simulink model "RADTRANS002"  (R2020b)
settings: Solver=VariableStepAuto  StartTime=0.0  StopTime=10.0  RelTol=1e-3
undefined symbols (not defined in the file): Line_110_C, Line_110_L, Line_110_R, Line_220_C, Line_220_L, Line_220_R, Line_35_C, Line_35_L, Line_35_R, Line_6_L, Line_6_R, Sys_f_Hz, Sys_V_net_kV, Tr_110_35_L_pu, Tr_110_35_R_pu, Tr_110_35_Sn_VA, Tr_110_35_V_HV_kV, Tr_110_35_V_LV_kV, Tr_110_6_L_pu, Tr_110_6_R_pu, Tr_110_6_Sn_VA, Tr_110_6_V_HV_kV, Tr_110_6_V_LV_kV, Tr_220_110_L_pu, Tr_220_110_R_pu, Tr_220_110_Sn_VA, Tr_220_110_V_HV_kV, Tr_220_110_V_LV_kV, Tr_35_04_L_pu, Tr_35_04_R_pu, Tr_35_04_Sn_VA, Tr_35_04_V_HV_kV, Tr_35_04_V_LV_kV, Tr_6_04_L_pu, Tr_6_04_R_pu, Tr_6_04_Sn_VA, Tr_6_04_V_HV_kV, Tr_6_04_V_LV_kV, Ts_powergui
libraries: dspstat3 x288, powerlib x202, powerlib_meascontrol x72
(part 5 of 7)

== system RADTRANS002/M_IN_Завод_6_1 ==
  Iptg_61 : Display
      settings: Format=bank
  PQptg_61 : Scope  NumInputPorts=2
  "Power0 (3ph, Instantaneous)" : powerlib_meascontrol/Measurements/Power (3ph, Instantaneous)
  Pptg_61 : Display
      settings: Format=bank
  Qptg_61 : Display
      settings: Format=bank
  RMS3 : dspstat3/RMS  run=off  directionMode=Each column  dimension=1  InputProcessing=Columns as channels (frame based)  reset_popup=None
  RMS4 : dspstat3/RMS  run=off  directionMode=Each column  dimension=1  InputProcessing=Columns as channels (frame based)  reset_popup=None
  RMS61 : dspstat3/RMS  run=off  directionMode=Each column  dimension=1  InputProcessing=Columns as channels (frame based)  reset_popup=None
  RMSpt_61 : dspstat3/RMS  run=off  directionMode=Each column  dimension=1  InputProcessing=Columns as channels (frame based)  reset_popup=None
  Real-Ima to Complex : RealImagToComplex
  S : Abs
  SSptg_61 : Scope
  Sptg_61 : Display
      settings: Format=bank
  Three-Phase V-I Measurementpt_61 : powerlib/Measurements/Three-Phase V-I Measurement  VoltageMeasurement=phase-to-ground  SetLabelV=off  LabelV=Vabc  Vpu=off  VpuLL=off  CurrentMeasurement=yes  SetLabelI=off  LabelI=Iabc  Ipu=off  Pbase=100e6  Vbase=500e3  OutputType=Complex  PhasorSimulation=off  PSBequivalent=0
  UIptg_61 : Scope  NumInputPorts=2
  Uptg_61 : Display
      settings: Format=bank
  a : PMIOPort  Side=Right
  b : PMIOPort  Port=2  Side=Right
  c : PMIOPort  Port=3  Side=Right
  A : PMIOPort  Port=4  Side=Left
  B : PMIOPort  Port=5  Side=Left
  C : PMIOPort  Port=6  Side=Left
  tag scope: I_ptg_61=global, P_ptg_61=global, Q_ptg_61=global, S_ptg_61=global, U_ptg_61=global
  wires:
  S/1 -> [S_ptg_61]
  Real-Ima to Complex/1 -> S/1
  [S_ptg_61] -> Sptg_61/1
  [S_ptg_61] -> SSptg_61/1
  [P_ptg_61] -> RMSpt_61/1
  RMSpt_61/1 -> Pptg_61/1
  RMS61/1 -> Qptg_61/1
  [U_ptg_61] -> RMS3/1
  RMS3/1 -> Uptg_61/1
  [P_ptg_61] -> Real-Ima to Complex/1
  [Q_ptg_61] -> RMS61/1
  [I_ptg_61] -> RMS4/1
  RMS4/1 -> Iptg_61/1
  [U_ptg_61] -> UIptg_61/1  "U"
  [P_ptg_61] -> PQptg_61/1  "P"
  [I_ptg_61] -> UIptg_61/2  "I"
  Three-Phase V-I Measurementpt_61/1 -> [U_ptg_61]
  [Q_ptg_61] -> Real-Ima to Complex/2
  Three-Phase V-I Measurementpt_61/2 -> [I_ptg_61]
  [U_ptg_61] -> "Power0 (3ph, Instantaneous)"/1
  [I_ptg_61] -> "Power0 (3ph, Instantaneous)"/2
  "Power0 (3ph, Instantaneous)"/2 -> [Q_ptg_61]
  "Power0 (3ph, Instantaneous)"/1 -> [P_ptg_61]
  [Q_ptg_61] -> PQptg_61/2  "Q"
  connections:
  Three-Phase V-I Measurementpt_61/LConn1 -- A/RConn1
  Three-Phase V-I Measurementpt_61/RConn1 -- a/RConn1
  Three-Phase V-I Measurementpt_61/LConn2 -- B/RConn1
  Three-Phase V-I Measurementpt_61/LConn3 -- C/RConn1
  Three-Phase V-I Measurementpt_61/RConn3 -- c/RConn1
  Three-Phase V-I Measurementpt_61/RConn2 -- b/RConn1

== system RADTRANS002/M_IN_Завод_6_2 ==
  Iptg_63 : Display
      settings: Format=bank
  PQptg_63 : Scope  NumInputPorts=2
  "Power0 (3ph, Instantaneous)" : powerlib_meascontrol/Measurements/Power (3ph, Instantaneous)
  Pptg_63 : Display
      settings: Format=bank
  Qptg_63 : Display
      settings: Format=bank
  RMS3 : dspstat3/RMS  run=off  directionMode=Each column  dimension=1  InputProcessing=Columns as channels (frame based)  reset_popup=None
  RMS4 : dspstat3/RMS  run=off  directionMode=Each column  dimension=1  InputProcessing=Columns as channels (frame based)  reset_popup=None
  RMS63 : dspstat3/RMS  run=off  directionMode=Each column  dimension=1  InputProcessing=Columns as channels (frame based)  reset_popup=None
  RMSpt_63 : dspstat3/RMS  run=off  directionMode=Each column  dimension=1  InputProcessing=Columns as channels (frame based)  reset_popup=None
  Real-Ima to Complex : RealImagToComplex
  S : Abs
  SSptg_63 : Scope
  Sptg_63 : Display
      settings: Format=bank
  Three-Phase V-I Measurementpt_63 : powerlib/Measurements/Three-Phase V-I Measurement  VoltageMeasurement=phase-to-ground  SetLabelV=off  LabelV=Vabc  Vpu=off  VpuLL=off  CurrentMeasurement=yes  SetLabelI=off  LabelI=Iabc  Ipu=off  Pbase=100e6  Vbase=500e3  OutputType=Complex  PhasorSimulation=off  PSBequivalent=0
  UIptg_63 : Scope  NumInputPorts=2
  Uptg_63 : Display
      settings: Format=bank
  a : PMIOPort  Side=Right
  b : PMIOPort  Port=2  Side=Right
  c : PMIOPort  Port=3  Side=Right
  A : PMIOPort  Port=4  Side=Left
  B : PMIOPort  Port=5  Side=Left
  C : PMIOPort  Port=6  Side=Left
  tag scope: I_ptg_63=global, P_ptg_63=global, Q_ptg_63=global, S_ptg_63=global, U_ptg_63=global
  wires:
  S/1 -> [S_ptg_63]
  Real-Ima to Complex/1 -> S/1
  [S_ptg_63] -> Sptg_63/1
  [S_ptg_63] -> SSptg_63/1
  [P_ptg_63] -> RMSpt_63/1
  RMSpt_63/1 -> Pptg_63/1
  RMS63/1 -> Qptg_63/1
  [U_ptg_63] -> RMS3/1
  RMS3/1 -> Uptg_63/1
  [P_ptg_63] -> Real-Ima to Complex/1
  [Q_ptg_63] -> RMS63/1
  [I_ptg_63] -> RMS4/1
  RMS4/1 -> Iptg_63/1
  [U_ptg_63] -> UIptg_63/1  "U"
  [P_ptg_63] -> PQptg_63/1  "P"
  [I_ptg_63] -> UIptg_63/2  "I"
  Three-Phase V-I Measurementpt_63/1 -> [U_ptg_63]
  [Q_ptg_63] -> Real-Ima to Complex/2
  Three-Phase V-I Measurementpt_63/2 -> [I_ptg_63]
  [U_ptg_63] -> "Power0 (3ph, Instantaneous)"/1
  [I_ptg_63] -> "Power0 (3ph, Instantaneous)"/2
  "Power0 (3ph, Instantaneous)"/2 -> [Q_ptg_63]
  "Power0 (3ph, Instantaneous)"/1 -> [P_ptg_63]
  [Q_ptg_63] -> PQptg_63/2  "Q"
  connections:
  Three-Phase V-I Measurementpt_63/LConn1 -- A/RConn1
  Three-Phase V-I Measurementpt_63/RConn1 -- a/RConn1
  Three-Phase V-I Measurementpt_63/LConn2 -- B/RConn1
  Three-Phase V-I Measurementpt_63/LConn3 -- C/RConn1
  Three-Phase V-I Measurementpt_63/RConn3 -- c/RConn1
  Three-Phase V-I Measurementpt_63/RConn2 -- b/RConn1

== system RADTRANS002/M_OUT_Город_1_1 ==
  Iptg_6 : Display
      settings: Format=bank
  PQptg_6 : Scope  NumInputPorts=2
  "Power0 (3ph, Instantaneous)" : powerlib_meascontrol/Measurements/Power (3ph, Instantaneous)
  Pptg_6 : Display
      settings: Format=bank
  Qptg_6 : Display
      settings: Format=bank
  RMS3 : dspstat3/RMS  run=off  directionMode=Each column  dimension=1  InputProcessing=Columns as channels (frame based)  reset_popup=None
  RMS4 : dspstat3/RMS  run=off  directionMode=Each column  dimension=1  InputProcessing=Columns as channels (frame based)  reset_popup=None
  RMS6 : dspstat3/RMS  run=off  directionMode=Each column  dimension=1  InputProcessing=Columns as channels (frame based)  reset_popup=None
  RMSpt_6 : dspstat3/RMS  run=off  directionMode=Each column  dimension=1  InputProcessing=Columns as channels (frame based)  reset_popup=None
  Real-Ima to Complex : RealImagToComplex
  S : Abs
  SSptg_6 : Scope
  Sptg_6 : Display
      settings: Format=bank
  Three-Phase V-I Measurementpt_6 : powerlib/Measurements/Three-Phase V-I Measurement  VoltageMeasurement=phase-to-ground  SetLabelV=off  LabelV=Vabc  Vpu=off  VpuLL=off  CurrentMeasurement=yes  SetLabelI=off  LabelI=Iabc  Ipu=off  Pbase=100e6  Vbase=500e3  OutputType=Complex  PhasorSimulation=off  PSBequivalent=0
  UIptg_6 : Scope  NumInputPorts=2
  Uptg_6 : Display
      settings: Format=bank
  a : PMIOPort  Side=Right
  b : PMIOPort  Port=2  Side=Right
  c : PMIOPort  Port=3  Side=Right
  A : PMIOPort  Port=4  Side=Left
  B : PMIOPort  Port=5  Side=Left
  C : PMIOPort  Port=6  Side=Left
  tag scope: I_ptg_6=global, P_ptg_6=global, Q_ptg_6=global, S_ptg_6=global, U_ptg_6=global
  wires:
  S/1 -> [S_ptg_6]
  Real-Ima to Complex/1 -> S/1
  [S_ptg_6] -> Sptg_6/1
  [S_ptg_6] -> SSptg_6/1
  [P_ptg_6] -> RMSpt_6/1
  RMSpt_6/1 -> Pptg_6/1
  RMS6/1 -> Qptg_6/1
  [U_ptg_6] -> RMS3/1
  RMS3/1 -> Uptg_6/1
  [P_ptg_6] -> Real-Ima to Complex/1
  [Q_ptg_6] -> RMS6/1
  [I_ptg_6] -> RMS4/1
  RMS4/1 -> Iptg_6/1
  [U_ptg_6] -> UIptg_6/1  "U"
  [P_ptg_6] -> PQptg_6/1  "P"
  [I_ptg_6] -> UIptg_6/2  "I"
  Three-Phase V-I Measurementpt_6/1 -> [U_ptg_6]
  [Q_ptg_6] -> Real-Ima to Complex/2
  Three-Phase V-I Measurementpt_6/2 -> [I_ptg_6]
  [U_ptg_6] -> "Power0 (3ph, Instantaneous)"/1
  [I_ptg_6] -> "Power0 (3ph, Instantaneous)"/2
  "Power0 (3ph, Instantaneous)"/2 -> [Q_ptg_6]
  "Power0 (3ph, Instantaneous)"/1 -> [P_ptg_6]
  [Q_ptg_6] -> PQptg_6/2  "Q"
  connections:
  Three-Phase V-I Measurementpt_6/LConn1 -- A/RConn1
  Three-Phase V-I Measurementpt_6/RConn1 -- a/RConn1
  Three-Phase V-I Measurementpt_6/LConn2 -- B/RConn1
  Three-Phase V-I Measurementpt_6/LConn3 -- C/RConn1
  Three-Phase V-I Measurementpt_6/RConn3 -- c/RConn1
  Three-Phase V-I Measurementpt_6/RConn2 -- b/RConn1

== system RADTRANS002/M_OUT_Город_1_2 ==
  Iptg_8 : Display
      settings: Format=bank
  PQptg_8 : Scope  NumInputPorts=2
  "Power0 (3ph, Instantaneous)" : powerlib_meascontrol/Measurements/Power (3ph, Instantaneous)
  Pptg_8 : Display
      settings: Format=bank
  Qptg_8 : Display
      settings: Format=bank
  RMS3 : dspstat3/RMS  run=off  directionMode=Each column  dimension=1  InputProcessing=Columns as channels (frame based)  reset_popup=None
  RMS4 : dspstat3/RMS  run=off  directionMode=Each column  dimension=1  InputProcessing=Columns as channels (frame based)  reset_popup=None
  RMS8 : dspstat3/RMS  run=off  directionMode=Each column  dimension=1  InputProcessing=Columns as channels (frame based)  reset_popup=None
  RMSpt_8 : dspstat3/RMS  run=off  directionMode=Each column  dimension=1  InputProcessing=Columns as channels (frame based)  reset_popup=None
  Real-Ima to Complex : RealImagToComplex
  S : Abs
  SSptg_8 : Scope
  Sptg_8 : Display
      settings: Format=bank
  Three-Phase V-I Measurementpt_8 : powerlib/Measurements/Three-Phase V-I Measurement  VoltageMeasurement=phase-to-ground  SetLabelV=off  LabelV=Vabc  Vpu=off  VpuLL=off  CurrentMeasurement=yes  SetLabelI=off  LabelI=Iabc  Ipu=off  Pbase=100e6  Vbase=500e3  OutputType=Complex  PhasorSimulation=off  PSBequivalent=0
  UIptg_8 : Scope  NumInputPorts=2
  Uptg_8 : Display
      settings: Format=bank
  a : PMIOPort  Side=Right
  b : PMIOPort  Port=2  Side=Right
  c : PMIOPort  Port=3  Side=Right
  A : PMIOPort  Port=4  Side=Left
  B : PMIOPort  Port=5  Side=Left
  C : PMIOPort  Port=6  Side=Left
  tag scope: I_ptg_8=global, P_ptg_8=global, Q_ptg_8=global, S_ptg_8=global, U_ptg_8=global
  wires:
  S/1 -> [S_ptg_8]
  Real-Ima to Complex/1 -> S/1
  [S_ptg_8] -> Sptg_8/1
  [S_ptg_8] -> SSptg_8/1
  [P_ptg_8] -> RMSpt_8/1
  RMSpt_8/1 -> Pptg_8/1
  RMS8/1 -> Qptg_8/1
  [U_ptg_8] -> RMS3/1
  RMS3/1 -> Uptg_8/1
  [P_ptg_8] -> Real-Ima to Complex/1
  [Q_ptg_8] -> RMS8/1
  [I_ptg_8] -> RMS4/1
  RMS4/1 -> Iptg_8/1
  [U_ptg_8] -> UIptg_8/1  "U"
  [P_ptg_8] -> PQptg_8/1  "P"
  [I_ptg_8] -> UIptg_8/2  "I"
  Three-Phase V-I Measurementpt_8/1 -> [U_ptg_8]
  [Q_ptg_8] -> Real-Ima to Complex/2
  Three-Phase V-I Measurementpt_8/2 -> [I_ptg_8]
  [U_ptg_8] -> "Power0 (3ph, Instantaneous)"/1
  [I_ptg_8] -> "Power0 (3ph, Instantaneous)"/2
  "Power0 (3ph, Instantaneous)"/2 -> [Q_ptg_8]
  "Power0 (3ph, Instantaneous)"/1 -> [P_ptg_8]
  [Q_ptg_8] -> PQptg_8/2  "Q"
  connections:
  Three-Phase V-I Measurementpt_8/LConn1 -- A/RConn1
  Three-Phase V-I Measurementpt_8/RConn1 -- a/RConn1
  Three-Phase V-I Measurementpt_8/LConn2 -- B/RConn1
  Three-Phase V-I Measurementpt_8/LConn3 -- C/RConn1
  Three-Phase V-I Measurementpt_8/RConn3 -- c/RConn1
  Three-Phase V-I Measurementpt_8/RConn2 -- b/RConn1

== system RADTRANS002/M_OUT_Город_1_3 ==
  Iptg_10 : Display
      settings: Format=bank
  PQptg_10 : Scope  NumInputPorts=2
  "Power0 (3ph, Instantaneous)" : powerlib_meascontrol/Measurements/Power (3ph, Instantaneous)
  Pptg_10 : Display
      settings: Format=bank
  Qptg_10 : Display
      settings: Format=bank
  RMS10 : dspstat3/RMS  run=off  directionMode=Each column  dimension=1  InputProcessing=Columns as channels (frame based)  reset_popup=None
  RMS3 : dspstat3/RMS  run=off  directionMode=Each column  dimension=1  InputProcessing=Columns as channels (frame based)  reset_popup=None
  RMS4 : dspstat3/RMS  run=off  directionMode=Each column  dimension=1  InputProcessing=Columns as channels (frame based)  reset_popup=None
  RMSpt_10 : dspstat3/RMS  run=off  directionMode=Each column  dimension=1  InputProcessing=Columns as channels (frame based)  reset_popup=None
  Real-Ima to Complex : RealImagToComplex
  S : Abs
  SSptg_10 : Scope
  Sptg_10 : Display
      settings: Format=bank
  Three-Phase V-I Measurementpt_10 : powerlib/Measurements/Three-Phase V-I Measurement  VoltageMeasurement=phase-to-ground  SetLabelV=off  LabelV=Vabc  Vpu=off  VpuLL=off  CurrentMeasurement=yes  SetLabelI=off  LabelI=Iabc  Ipu=off  Pbase=100e6  Vbase=500e3  OutputType=Complex  PhasorSimulation=off  PSBequivalent=0
  UIptg_10 : Scope  NumInputPorts=2
  Uptg_10 : Display
      settings: Format=bank
  a : PMIOPort  Side=Right
  b : PMIOPort  Port=2  Side=Right
  c : PMIOPort  Port=3  Side=Right
  A : PMIOPort  Port=4  Side=Left
  B : PMIOPort  Port=5  Side=Left
  C : PMIOPort  Port=6  Side=Left
  tag scope: I_ptg_10=global, P_ptg_10=global, Q_ptg_10=global, S_ptg_10=global, U_ptg_10=global
  wires:
  S/1 -> [S_ptg_10]
  Real-Ima to Complex/1 -> S/1
  [S_ptg_10] -> Sptg_10/1
  [S_ptg_10] -> SSptg_10/1
  [P_ptg_10] -> RMSpt_10/1
  RMSpt_10/1 -> Pptg_10/1
  RMS10/1 -> Qptg_10/1
  [U_ptg_10] -> RMS3/1
  RMS3/1 -> Uptg_10/1
  [P_ptg_10] -> Real-Ima to Complex/1
  [Q_ptg_10] -> RMS10/1
  [I_ptg_10] -> RMS4/1
  RMS4/1 -> Iptg_10/1
  [U_ptg_10] -> UIptg_10/1  "U"
  [P_ptg_10] -> PQptg_10/1  "P"
  [I_ptg_10] -> UIptg_10/2  "I"
  Three-Phase V-I Measurementpt_10/1 -> [U_ptg_10]
  [Q_ptg_10] -> Real-Ima to Complex/2
  Three-Phase V-I Measurementpt_10/2 -> [I_ptg_10]
  [U_ptg_10] -> "Power0 (3ph, Instantaneous)"/1
  [I_ptg_10] -> "Power0 (3ph, Instantaneous)"/2
  "Power0 (3ph, Instantaneous)"/2 -> [Q_ptg_10]
  "Power0 (3ph, Instantaneous)"/1 -> [P_ptg_10]
  [Q_ptg_10] -> PQptg_10/2  "Q"
  connections:
  Three-Phase V-I Measurementpt_10/LConn1 -- A/RConn1
  Three-Phase V-I Measurementpt_10/RConn1 -- a/RConn1
  Three-Phase V-I Measurementpt_10/LConn2 -- B/RConn1
  Three-Phase V-I Measurementpt_10/LConn3 -- C/RConn1
  Three-Phase V-I Measurementpt_10/RConn3 -- c/RConn1
  Three-Phase V-I Measurementpt_10/RConn2 -- b/RConn1

== system RADTRANS002/M_OUT_Город_1_4 ==
  Iptg_12 : Display
      settings: Format=bank
  PQptg_12 : Scope  NumInputPorts=2
  "Power0 (3ph, Instantaneous)" : powerlib_meascontrol/Measurements/Power (3ph, Instantaneous)
  Pptg_12 : Display
      settings: Format=bank
  Qptg_12 : Display
      settings: Format=bank
  RMS12 : dspstat3/RMS  run=off  directionMode=Each column  dimension=1  InputProcessing=Columns as channels (frame based)  reset_popup=None
  RMS3 : dspstat3/RMS  run=off  directionMode=Each column  dimension=1  InputProcessing=Columns as channels (frame based)  reset_popup=None
  RMS4 : dspstat3/RMS  run=off  directionMode=Each column  dimension=1  InputProcessing=Columns as channels (frame based)  reset_popup=None
  RMSpt_12 : dspstat3/RMS  run=off  directionMode=Each column  dimension=1  InputProcessing=Columns as channels (frame based)  reset_popup=None
  Real-Ima to Complex : RealImagToComplex
  S : Abs
  SSptg_12 : Scope
  Sptg_12 : Display
      settings: Format=bank
  Three-Phase V-I Measurementpt_12 : powerlib/Measurements/Three-Phase V-I Measurement  VoltageMeasurement=phase-to-ground  SetLabelV=off  LabelV=Vabc  Vpu=off  VpuLL=off  CurrentMeasurement=yes  SetLabelI=off  LabelI=Iabc  Ipu=off  Pbase=100e6  Vbase=500e3  OutputType=Complex  PhasorSimulation=off  PSBequivalent=0
  UIptg_12 : Scope  NumInputPorts=2
  Uptg_12 : Display
      settings: Format=bank
  a : PMIOPort  Side=Right
  b : PMIOPort  Port=2  Side=Right
  c : PMIOPort  Port=3  Side=Right
  A : PMIOPort  Port=4  Side=Left
  B : PMIOPort  Port=5  Side=Left
  C : PMIOPort  Port=6  Side=Left
  tag scope: I_ptg_12=global, P_ptg_12=global, Q_ptg_12=global, S_ptg_12=global, U_ptg_12=global
  wires:
  S/1 -> [S_ptg_12]
  Real-Ima to Complex/1 -> S/1
  [S_ptg_12] -> Sptg_12/1
  [S_ptg_12] -> SSptg_12/1
  [P_ptg_12] -> RMSpt_12/1
  RMSpt_12/1 -> Pptg_12/1
  RMS12/1 -> Qptg_12/1
  [U_ptg_12] -> RMS3/1
  RMS3/1 -> Uptg_12/1
  [P_ptg_12] -> Real-Ima to Complex/1
  [Q_ptg_12] -> RMS12/1
  [I_ptg_12] -> RMS4/1
  RMS4/1 -> Iptg_12/1
  [U_ptg_12] -> UIptg_12/1  "U"
  [P_ptg_12] -> PQptg_12/1  "P"
  [I_ptg_12] -> UIptg_12/2  "I"
  Three-Phase V-I Measurementpt_12/1 -> [U_ptg_12]
  [Q_ptg_12] -> Real-Ima to Complex/2
  Three-Phase V-I Measurementpt_12/2 -> [I_ptg_12]
  [U_ptg_12] -> "Power0 (3ph, Instantaneous)"/1
  [I_ptg_12] -> "Power0 (3ph, Instantaneous)"/2
  "Power0 (3ph, Instantaneous)"/2 -> [Q_ptg_12]
  "Power0 (3ph, Instantaneous)"/1 -> [P_ptg_12]
  [Q_ptg_12] -> PQptg_12/2  "Q"
  connections:
  Three-Phase V-I Measurementpt_12/LConn1 -- A/RConn1
  Three-Phase V-I Measurementpt_12/RConn1 -- a/RConn1
  Three-Phase V-I Measurementpt_12/LConn2 -- B/RConn1
  Three-Phase V-I Measurementpt_12/LConn3 -- C/RConn1
  Three-Phase V-I Measurementpt_12/RConn3 -- c/RConn1
  Three-Phase V-I Measurementpt_12/RConn2 -- b/RConn1

== system RADTRANS002/M_OUT_Город_2_1 ==
  Iptg_18 : Display
      settings: Format=bank
  PQptg_18 : Scope  NumInputPorts=2
  "Power0 (3ph, Instantaneous)" : powerlib_meascontrol/Measurements/Power (3ph, Instantaneous)
  Pptg_18 : Display
      settings: Format=bank
  Qptg_18 : Display
      settings: Format=bank
  RMS18 : dspstat3/RMS  run=off  directionMode=Each column  dimension=1  InputProcessing=Columns as channels (frame based)  reset_popup=None
  RMS3 : dspstat3/RMS  run=off  directionMode=Each column  dimension=1  InputProcessing=Columns as channels (frame based)  reset_popup=None
  RMS4 : dspstat3/RMS  run=off  directionMode=Each column  dimension=1  InputProcessing=Columns as channels (frame based)  reset_popup=None
  RMSpt_18 : dspstat3/RMS  run=off  directionMode=Each column  dimension=1  InputProcessing=Columns as channels (frame based)  reset_popup=None
  Real-Ima to Complex : RealImagToComplex
  S : Abs
  SSptg_18 : Scope
  Sptg_18 : Display
      settings: Format=bank
  Three-Phase V-I Measurementpt_18 : powerlib/Measurements/Three-Phase V-I Measurement  VoltageMeasurement=phase-to-ground  SetLabelV=off  LabelV=Vabc  Vpu=off  VpuLL=off  CurrentMeasurement=yes  SetLabelI=off  LabelI=Iabc  Ipu=off  Pbase=100e6  Vbase=500e3  OutputType=Complex  PhasorSimulation=off  PSBequivalent=0
  UIptg_18 : Scope  NumInputPorts=2
  Uptg_18 : Display
      settings: Format=bank
  a : PMIOPort  Side=Right
  b : PMIOPort  Port=2  Side=Right
  c : PMIOPort  Port=3  Side=Right
  A : PMIOPort  Port=4  Side=Left
  B : PMIOPort  Port=5  Side=Left
  C : PMIOPort  Port=6  Side=Left
  tag scope: I_ptg_18=global, P_ptg_18=global, Q_ptg_18=global, S_ptg_18=global, U_ptg_18=global
  wires:
  S/1 -> [S_ptg_18]
  Real-Ima to Complex/1 -> S/1
  [S_ptg_18] -> Sptg_18/1
  [S_ptg_18] -> SSptg_18/1
  [P_ptg_18] -> RMSpt_18/1
  RMSpt_18/1 -> Pptg_18/1
  RMS18/1 -> Qptg_18/1
  [U_ptg_18] -> RMS3/1
  RMS3/1 -> Uptg_18/1
  [P_ptg_18] -> Real-Ima to Complex/1
  [Q_ptg_18] -> RMS18/1
  [I_ptg_18] -> RMS4/1
  RMS4/1 -> Iptg_18/1
  [U_ptg_18] -> UIptg_18/1  "U"
  [P_ptg_18] -> PQptg_18/1  "P"
  [I_ptg_18] -> UIptg_18/2  "I"
  Three-Phase V-I Measurementpt_18/1 -> [U_ptg_18]
  [Q_ptg_18] -> Real-Ima to Complex/2
  Three-Phase V-I Measurementpt_18/2 -> [I_ptg_18]
  [U_ptg_18] -> "Power0 (3ph, Instantaneous)"/1
  [I_ptg_18] -> "Power0 (3ph, Instantaneous)"/2
  "Power0 (3ph, Instantaneous)"/2 -> [Q_ptg_18]
  "Power0 (3ph, Instantaneous)"/1 -> [P_ptg_18]
  [Q_ptg_18] -> PQptg_18/2  "Q"
  connections:
  Three-Phase V-I Measurementpt_18/LConn1 -- A/RConn1
  Three-Phase V-I Measurementpt_18/RConn1 -- a/RConn1
  Three-Phase V-I Measurementpt_18/LConn2 -- B/RConn1
  Three-Phase V-I Measurementpt_18/LConn3 -- C/RConn1
  Three-Phase V-I Measurementpt_18/RConn3 -- c/RConn1
  Three-Phase V-I Measurementpt_18/RConn2 -- b/RConn1

== system RADTRANS002/M_OUT_Город_2_2 ==
  Iptg_20 : Display
      settings: Format=bank
  PQptg_20 : Scope  NumInputPorts=2
  "Power0 (3ph, Instantaneous)" : powerlib_meascontrol/Measurements/Power (3ph, Instantaneous)
  Pptg_20 : Display
      settings: Format=bank
  Qptg_20 : Display
      settings: Format=bank
  RMS20 : dspstat3/RMS  run=off  directionMode=Each column  dimension=1  InputProcessing=Columns as channels (frame based)  reset_popup=None
  RMS3 : dspstat3/RMS  run=off  directionMode=Each column  dimension=1  InputProcessing=Columns as channels (frame based)  reset_popup=None
  RMS4 : dspstat3/RMS  run=off  directionMode=Each column  dimension=1  InputProcessing=Columns as channels (frame based)  reset_popup=None
  RMSpt_20 : dspstat3/RMS  run=off  directionMode=Each column  dimension=1  InputProcessing=Columns as channels (frame based)  reset_popup=None
  Real-Ima to Complex : RealImagToComplex
  S : Abs
  SSptg_20 : Scope
  Sptg_20 : Display
      settings: Format=bank
  Three-Phase V-I Measurementpt_20 : powerlib/Measurements/Three-Phase V-I Measurement  VoltageMeasurement=phase-to-ground  SetLabelV=off  LabelV=Vabc  Vpu=off  VpuLL=off  CurrentMeasurement=yes  SetLabelI=off  LabelI=Iabc  Ipu=off  Pbase=100e6  Vbase=500e3  OutputType=Complex  PhasorSimulation=off  PSBequivalent=0
  UIptg_20 : Scope  NumInputPorts=2
  Uptg_20 : Display
      settings: Format=bank
  a : PMIOPort  Side=Right
  b : PMIOPort  Port=2  Side=Right
  c : PMIOPort  Port=3  Side=Right
  A : PMIOPort  Port=4  Side=Left
  B : PMIOPort  Port=5  Side=Left
  C : PMIOPort  Port=6  Side=Left
  tag scope: I_ptg_20=global, P_ptg_20=global, Q_ptg_20=global, S_ptg_20=global, U_ptg_20=global
  wires:
  S/1 -> [S_ptg_20]
  Real-Ima to Complex/1 -> S/1
  [S_ptg_20] -> Sptg_20/1
  [S_ptg_20] -> SSptg_20/1
  [P_ptg_20] -> RMSpt_20/1
  RMSpt_20/1 -> Pptg_20/1
  RMS20/1 -> Qptg_20/1
  [U_ptg_20] -> RMS3/1
  RMS3/1 -> Uptg_20/1
  [P_ptg_20] -> Real-Ima to Complex/1
  [Q_ptg_20] -> RMS20/1
  [I_ptg_20] -> RMS4/1
  RMS4/1 -> Iptg_20/1
  [U_ptg_20] -> UIptg_20/1  "U"
  [P_ptg_20] -> PQptg_20/1  "P"
  [I_ptg_20] -> UIptg_20/2  "I"
  Three-Phase V-I Measurementpt_20/1 -> [U_ptg_20]
  [Q_ptg_20] -> Real-Ima to Complex/2
  Three-Phase V-I Measurementpt_20/2 -> [I_ptg_20]
  [U_ptg_20] -> "Power0 (3ph, Instantaneous)"/1
  [I_ptg_20] -> "Power0 (3ph, Instantaneous)"/2
  "Power0 (3ph, Instantaneous)"/2 -> [Q_ptg_20]
  "Power0 (3ph, Instantaneous)"/1 -> [P_ptg_20]
  [Q_ptg_20] -> PQptg_20/2  "Q"
  connections:
  Three-Phase V-I Measurementpt_20/LConn1 -- A/RConn1
  Three-Phase V-I Measurementpt_20/RConn1 -- a/RConn1
  Three-Phase V-I Measurementpt_20/LConn2 -- B/RConn1
  Three-Phase V-I Measurementpt_20/LConn3 -- C/RConn1
  Three-Phase V-I Measurementpt_20/RConn3 -- c/RConn1
  Three-Phase V-I Measurementpt_20/RConn2 -- b/RConn1

== system RADTRANS002/M_OUT_Город_2_3 ==
  Iptg_22 : Display
      settings: Format=bank
  PQptg_22 : Scope  NumInputPorts=2
  "Power0 (3ph, Instantaneous)" : powerlib_meascontrol/Measurements/Power (3ph, Instantaneous)
  Pptg_22 : Display
      settings: Format=bank
  Qptg_22 : Display
      settings: Format=bank
  RMS22 : dspstat3/RMS  run=off  directionMode=Each column  dimension=1  InputProcessing=Columns as channels (frame based)  reset_popup=None
  RMS3 : dspstat3/RMS  run=off  directionMode=Each column  dimension=1  InputProcessing=Columns as channels (frame based)  reset_popup=None
  RMS4 : dspstat3/RMS  run=off  directionMode=Each column  dimension=1  InputProcessing=Columns as channels (frame based)  reset_popup=None
  RMSpt_22 : dspstat3/RMS  run=off  directionMode=Each column  dimension=1  InputProcessing=Columns as channels (frame based)  reset_popup=None
  Real-Ima to Complex : RealImagToComplex
  S : Abs
  SSptg_22 : Scope
  Sptg_22 : Display
      settings: Format=bank
  Three-Phase V-I Measurementpt_22 : powerlib/Measurements/Three-Phase V-I Measurement  VoltageMeasurement=phase-to-ground  SetLabelV=off  LabelV=Vabc  Vpu=off  VpuLL=off  CurrentMeasurement=yes  SetLabelI=off  LabelI=Iabc  Ipu=off  Pbase=100e6  Vbase=500e3  OutputType=Complex  PhasorSimulation=off  PSBequivalent=0
  UIptg_22 : Scope  NumInputPorts=2
  Uptg_22 : Display
      settings: Format=bank
  a : PMIOPort  Side=Right
  b : PMIOPort  Port=2  Side=Right
  c : PMIOPort  Port=3  Side=Right
  A : PMIOPort  Port=4  Side=Left
  B : PMIOPort  Port=5  Side=Left
  C : PMIOPort  Port=6  Side=Left
  tag scope: I_ptg_22=global, P_ptg_22=global, Q_ptg_22=global, S_ptg_22=global, U_ptg_22=global
  wires:
  S/1 -> [S_ptg_22]
  Real-Ima to Complex/1 -> S/1
  [S_ptg_22] -> Sptg_22/1
  [S_ptg_22] -> SSptg_22/1
  [P_ptg_22] -> RMSpt_22/1
  RMSpt_22/1 -> Pptg_22/1
  RMS22/1 -> Qptg_22/1
  [U_ptg_22] -> RMS3/1
  RMS3/1 -> Uptg_22/1
  [P_ptg_22] -> Real-Ima to Complex/1
  [Q_ptg_22] -> RMS22/1
  [I_ptg_22] -> RMS4/1
  RMS4/1 -> Iptg_22/1
  [U_ptg_22] -> UIptg_22/1  "U"
  [P_ptg_22] -> PQptg_22/1  "P"
  [I_ptg_22] -> UIptg_22/2  "I"
  Three-Phase V-I Measurementpt_22/1 -> [U_ptg_22]
  [Q_ptg_22] -> Real-Ima to Complex/2
  Three-Phase V-I Measurementpt_22/2 -> [I_ptg_22]
  [U_ptg_22] -> "Power0 (3ph, Instantaneous)"/1
  [I_ptg_22] -> "Power0 (3ph, Instantaneous)"/2
  "Power0 (3ph, Instantaneous)"/2 -> [Q_ptg_22]
  "Power0 (3ph, Instantaneous)"/1 -> [P_ptg_22]
  [Q_ptg_22] -> PQptg_22/2  "Q"
  connections:
  Three-Phase V-I Measurementpt_22/LConn1 -- A/RConn1
  Three-Phase V-I Measurementpt_22/RConn1 -- a/RConn1
  Three-Phase V-I Measurementpt_22/LConn2 -- B/RConn1
  Three-Phase V-I Measurementpt_22/LConn3 -- C/RConn1
  Three-Phase V-I Measurementpt_22/RConn3 -- c/RConn1
  Three-Phase V-I Measurementpt_22/RConn2 -- b/RConn1

== system RADTRANS002/M_OUT_Город_2_4 ==
  Iptg_24 : Display
      settings: Format=bank
  PQptg_24 : Scope  NumInputPorts=2
  "Power0 (3ph, Instantaneous)" : powerlib_meascontrol/Measurements/Power (3ph, Instantaneous)
  Pptg_24 : Display
      settings: Format=bank
  Qptg_24 : Display
      settings: Format=bank
  RMS24 : dspstat3/RMS  run=off  directionMode=Each column  dimension=1  InputProcessing=Columns as channels (frame based)  reset_popup=None
  RMS3 : dspstat3/RMS  run=off  directionMode=Each column  dimension=1  InputProcessing=Columns as channels (frame based)  reset_popup=None
  RMS4 : dspstat3/RMS  run=off  directionMode=Each column  dimension=1  InputProcessing=Columns as channels (frame based)  reset_popup=None
  RMSpt_24 : dspstat3/RMS  run=off  directionMode=Each column  dimension=1  InputProcessing=Columns as channels (frame based)  reset_popup=None
  Real-Ima to Complex : RealImagToComplex
  S : Abs
  SSptg_24 : Scope
  Sptg_24 : Display
      settings: Format=bank
  Three-Phase V-I Measurementpt_24 : powerlib/Measurements/Three-Phase V-I Measurement  VoltageMeasurement=phase-to-ground  SetLabelV=off  LabelV=Vabc  Vpu=off  VpuLL=off  CurrentMeasurement=yes  SetLabelI=off  LabelI=Iabc  Ipu=off  Pbase=100e6  Vbase=500e3  OutputType=Complex  PhasorSimulation=off  PSBequivalent=0
  UIptg_24 : Scope  NumInputPorts=2
  Uptg_24 : Display
      settings: Format=bank
  a : PMIOPort  Side=Right
  b : PMIOPort  Port=2  Side=Right
  c : PMIOPort  Port=3  Side=Right
  A : PMIOPort  Port=4  Side=Left
  B : PMIOPort  Port=5  Side=Left
  C : PMIOPort  Port=6  Side=Left
  tag scope: I_ptg_24=global, P_ptg_24=global, Q_ptg_24=global, S_ptg_24=global, U_ptg_24=global
  wires:
  S/1 -> [S_ptg_24]
  Real-Ima to Complex/1 -> S/1
  [S_ptg_24] -> Sptg_24/1
  [S_ptg_24] -> SSptg_24/1
  [P_ptg_24] -> RMSpt_24/1
  RMSpt_24/1 -> Pptg_24/1
  RMS24/1 -> Qptg_24/1
  [U_ptg_24] -> RMS3/1
  RMS3/1 -> Uptg_24/1
  [P_ptg_24] -> Real-Ima to Complex/1
  [Q_ptg_24] -> RMS24/1
  [I_ptg_24] -> RMS4/1
  RMS4/1 -> Iptg_24/1
  [U_ptg_24] -> UIptg_24/1  "U"
  [P_ptg_24] -> PQptg_24/1  "P"
  [I_ptg_24] -> UIptg_24/2  "I"
  Three-Phase V-I Measurementpt_24/1 -> [U_ptg_24]
  [Q_ptg_24] -> Real-Ima to Complex/2
  Three-Phase V-I Measurementpt_24/2 -> [I_ptg_24]
  [U_ptg_24] -> "Power0 (3ph, Instantaneous)"/1
  [I_ptg_24] -> "Power0 (3ph, Instantaneous)"/2
  "Power0 (3ph, Instantaneous)"/2 -> [Q_ptg_24]
  "Power0 (3ph, Instantaneous)"/1 -> [P_ptg_24]
  [Q_ptg_24] -> PQptg_24/2  "Q"
  connections:
  Three-Phase V-I Measurementpt_24/LConn1 -- A/RConn1
  Three-Phase V-I Measurementpt_24/RConn1 -- a/RConn1
  Three-Phase V-I Measurementpt_24/LConn2 -- B/RConn1
  Three-Phase V-I Measurementpt_24/LConn3 -- C/RConn1
  Three-Phase V-I Measurementpt_24/RConn3 -- c/RConn1
  Three-Phase V-I Measurementpt_24/RConn2 -- b/RConn1

== system RADTRANS002/M_OUT_Город_3_1 ==
  Iptg_30 : Display
      settings: Format=bank
  PQptg_30 : Scope  NumInputPorts=2
  "Power0 (3ph, Instantaneous)" : powerlib_meascontrol/Measurements/Power (3ph, Instantaneous)
  Pptg_30 : Display
      settings: Format=bank
  Qptg_30 : Display
      settings: Format=bank
  RMS3 : dspstat3/RMS  run=off  directionMode=Each column  dimension=1  InputProcessing=Columns as channels (frame based)  reset_popup=None
  RMS30 : dspstat3/RMS  run=off  directionMode=Each column  dimension=1  InputProcessing=Columns as channels (frame based)  reset_popup=None
  RMS4 : dspstat3/RMS  run=off  directionMode=Each column  dimension=1  InputProcessing=Columns as channels (frame based)  reset_popup=None
  RMSpt_30 : dspstat3/RMS  run=off  directionMode=Each column  dimension=1  InputProcessing=Columns as channels (frame based)  reset_popup=None
  Real-Ima to Complex : RealImagToComplex
  S : Abs
  SSptg_30 : Scope
  Sptg_30 : Display
      settings: Format=bank
  Three-Phase V-I Measurementpt_30 : powerlib/Measurements/Three-Phase V-I Measurement  VoltageMeasurement=phase-to-ground  SetLabelV=off  LabelV=Vabc  Vpu=off  VpuLL=off  CurrentMeasurement=yes  SetLabelI=off  LabelI=Iabc  Ipu=off  Pbase=100e6  Vbase=500e3  OutputType=Complex  PhasorSimulation=off  PSBequivalent=0
  UIptg_30 : Scope  NumInputPorts=2
  Uptg_30 : Display
      settings: Format=bank
  a : PMIOPort  Side=Right
  b : PMIOPort  Port=2  Side=Right
  c : PMIOPort  Port=3  Side=Right
  A : PMIOPort  Port=4  Side=Left
  B : PMIOPort  Port=5  Side=Left
  C : PMIOPort  Port=6  Side=Left
  tag scope: I_ptg_30=global, P_ptg_30=global, Q_ptg_30=global, S_ptg_30=global, U_ptg_30=global
  wires:
  S/1 -> [S_ptg_30]
  Real-Ima to Complex/1 -> S/1
  [S_ptg_30] -> Sptg_30/1
  [S_ptg_30] -> SSptg_30/1
  [P_ptg_30] -> RMSpt_30/1
  RMSpt_30/1 -> Pptg_30/1
  RMS30/1 -> Qptg_30/1
  [U_ptg_30] -> RMS3/1
  RMS3/1 -> Uptg_30/1
  [P_ptg_30] -> Real-Ima to Complex/1
  [Q_ptg_30] -> RMS30/1
  [I_ptg_30] -> RMS4/1
  RMS4/1 -> Iptg_30/1
  [U_ptg_30] -> UIptg_30/1  "U"
  [P_ptg_30] -> PQptg_30/1  "P"
  [I_ptg_30] -> UIptg_30/2  "I"
  Three-Phase V-I Measurementpt_30/1 -> [U_ptg_30]
  [Q_ptg_30] -> Real-Ima to Complex/2
  Three-Phase V-I Measurementpt_30/2 -> [I_ptg_30]
  [U_ptg_30] -> "Power0 (3ph, Instantaneous)"/1
  [I_ptg_30] -> "Power0 (3ph, Instantaneous)"/2
  "Power0 (3ph, Instantaneous)"/2 -> [Q_ptg_30]
  "Power0 (3ph, Instantaneous)"/1 -> [P_ptg_30]
  [Q_ptg_30] -> PQptg_30/2  "Q"
  connections:
  Three-Phase V-I Measurementpt_30/LConn1 -- A/RConn1
  Three-Phase V-I Measurementpt_30/RConn1 -- a/RConn1
  Three-Phase V-I Measurementpt_30/LConn2 -- B/RConn1
  Three-Phase V-I Measurementpt_30/LConn3 -- C/RConn1
  Three-Phase V-I Measurementpt_30/RConn3 -- c/RConn1
  Three-Phase V-I Measurementpt_30/RConn2 -- b/RConn1

== system RADTRANS002/M_OUT_Город_3_2 ==
  Iptg_32 : Display
      settings: Format=bank
  PQptg_32 : Scope  NumInputPorts=2
  "Power0 (3ph, Instantaneous)" : powerlib_meascontrol/Measurements/Power (3ph, Instantaneous)
  Pptg_32 : Display
      settings: Format=bank
  Qptg_32 : Display
      settings: Format=bank
  RMS3 : dspstat3/RMS  run=off  directionMode=Each column  dimension=1  InputProcessing=Columns as channels (frame based)  reset_popup=None
  RMS32 : dspstat3/RMS  run=off  directionMode=Each column  dimension=1  InputProcessing=Columns as channels (frame based)  reset_popup=None
  RMS4 : dspstat3/RMS  run=off  directionMode=Each column  dimension=1  InputProcessing=Columns as channels (frame based)  reset_popup=None
  RMSpt_32 : dspstat3/RMS  run=off  directionMode=Each column  dimension=1  InputProcessing=Columns as channels (frame based)  reset_popup=None
  Real-Ima to Complex : RealImagToComplex
  S : Abs
  SSptg_32 : Scope
  Sptg_32 : Display
      settings: Format=bank
  Three-Phase V-I Measurementpt_32 : powerlib/Measurements/Three-Phase V-I Measurement  VoltageMeasurement=phase-to-ground  SetLabelV=off  LabelV=Vabc  Vpu=off  VpuLL=off  CurrentMeasurement=yes  SetLabelI=off  LabelI=Iabc  Ipu=off  Pbase=100e6  Vbase=500e3  OutputType=Complex  PhasorSimulation=off  PSBequivalent=0
  UIptg_32 : Scope  NumInputPorts=2
  Uptg_32 : Display
      settings: Format=bank
  a : PMIOPort  Side=Right
  b : PMIOPort  Port=2  Side=Right
  c : PMIOPort  Port=3  Side=Right
  A : PMIOPort  Port=4  Side=Left
  B : PMIOPort  Port=5  Side=Left
  C : PMIOPort  Port=6  Side=Left
  tag scope: I_ptg_32=global, P_ptg_32=global, Q_ptg_32=global, S_ptg_32=global, U_ptg_32=global
  wires:
  S/1 -> [S_ptg_32]
  Real-Ima to Complex/1 -> S/1
  [S_ptg_32] -> Sptg_32/1
  [S_ptg_32] -> SSptg_32/1
  [P_ptg_32] -> RMSpt_32/1
  RMSpt_32/1 -> Pptg_32/1
  RMS32/1 -> Qptg_32/1
  [U_ptg_32] -> RMS3/1
  RMS3/1 -> Uptg_32/1
  [P_ptg_32] -> Real-Ima to Complex/1
  [Q_ptg_32] -> RMS32/1
  [I_ptg_32] -> RMS4/1
  RMS4/1 -> Iptg_32/1
  [U_ptg_32] -> UIptg_32/1  "U"
  [P_ptg_32] -> PQptg_32/1  "P"
  [I_ptg_32] -> UIptg_32/2  "I"
  Three-Phase V-I Measurementpt_32/1 -> [U_ptg_32]
  [Q_ptg_32] -> Real-Ima to Complex/2
  Three-Phase V-I Measurementpt_32/2 -> [I_ptg_32]
  [U_ptg_32] -> "Power0 (3ph, Instantaneous)"/1
  [I_ptg_32] -> "Power0 (3ph, Instantaneous)"/2
  "Power0 (3ph, Instantaneous)"/2 -> [Q_ptg_32]
  "Power0 (3ph, Instantaneous)"/1 -> [P_ptg_32]
  [Q_ptg_32] -> PQptg_32/2  "Q"
  connections:
  Three-Phase V-I Measurementpt_32/LConn1 -- A/RConn1
  Three-Phase V-I Measurementpt_32/RConn1 -- a/RConn1
  Three-Phase V-I Measurementpt_32/LConn2 -- B/RConn1
  Three-Phase V-I Measurementpt_32/LConn3 -- C/RConn1
  Three-Phase V-I Measurementpt_32/RConn3 -- c/RConn1
  Three-Phase V-I Measurementpt_32/RConn2 -- b/RConn1

== system RADTRANS002/M_OUT_Город_3_3 ==
  Iptg_34 : Display
      settings: Format=bank
  PQptg_34 : Scope  NumInputPorts=2
  "Power0 (3ph, Instantaneous)" : powerlib_meascontrol/Measurements/Power (3ph, Instantaneous)
  Pptg_34 : Display
      settings: Format=bank
  Qptg_34 : Display
      settings: Format=bank
  RMS3 : dspstat3/RMS  run=off  directionMode=Each column  dimension=1  InputProcessing=Columns as channels (frame based)  reset_popup=None
  RMS34 : dspstat3/RMS  run=off  directionMode=Each column  dimension=1  InputProcessing=Columns as channels (frame based)  reset_popup=None
  RMS4 : dspstat3/RMS  run=off  directionMode=Each column  dimension=1  InputProcessing=Columns as channels (frame based)  reset_popup=None
  RMSpt_34 : dspstat3/RMS  run=off  directionMode=Each column  dimension=1  InputProcessing=Columns as channels (frame based)  reset_popup=None
  Real-Ima to Complex : RealImagToComplex
  S : Abs
  SSptg_34 : Scope
  Sptg_34 : Display
      settings: Format=bank
  Three-Phase V-I Measurementpt_34 : powerlib/Measurements/Three-Phase V-I Measurement  VoltageMeasurement=phase-to-ground  SetLabelV=off  LabelV=Vabc  Vpu=off  VpuLL=off  CurrentMeasurement=yes  SetLabelI=off  LabelI=Iabc  Ipu=off  Pbase=100e6  Vbase=500e3  OutputType=Complex  PhasorSimulation=off  PSBequivalent=0
  UIptg_34 : Scope  NumInputPorts=2
  Uptg_34 : Display
      settings: Format=bank
  a : PMIOPort  Side=Right
  b : PMIOPort  Port=2  Side=Right
  c : PMIOPort  Port=3  Side=Right
  A : PMIOPort  Port=4  Side=Left
  B : PMIOPort  Port=5  Side=Left
  C : PMIOPort  Port=6  Side=Left
  tag scope: I_ptg_34=global, P_ptg_34=global, Q_ptg_34=global, S_ptg_34=global, U_ptg_34=global
  wires:
  S/1 -> [S_ptg_34]
  Real-Ima to Complex/1 -> S/1
  [S_ptg_34] -> Sptg_34/1
  [S_ptg_34] -> SSptg_34/1
  [P_ptg_34] -> RMSpt_34/1
  RMSpt_34/1 -> Pptg_34/1
  RMS34/1 -> Qptg_34/1
  [U_ptg_34] -> RMS3/1
  RMS3/1 -> Uptg_34/1
  [P_ptg_34] -> Real-Ima to Complex/1
  [Q_ptg_34] -> RMS34/1
  [I_ptg_34] -> RMS4/1
  RMS4/1 -> Iptg_34/1
  [U_ptg_34] -> UIptg_34/1  "U"
  [P_ptg_34] -> PQptg_34/1  "P"
  [I_ptg_34] -> UIptg_34/2  "I"
  Three-Phase V-I Measurementpt_34/1 -> [U_ptg_34]
  [Q_ptg_34] -> Real-Ima to Complex/2
  Three-Phase V-I Measurementpt_34/2 -> [I_ptg_34]
  [U_ptg_34] -> "Power0 (3ph, Instantaneous)"/1
  [I_ptg_34] -> "Power0 (3ph, Instantaneous)"/2
  "Power0 (3ph, Instantaneous)"/2 -> [Q_ptg_34]
  "Power0 (3ph, Instantaneous)"/1 -> [P_ptg_34]
  [Q_ptg_34] -> PQptg_34/2  "Q"
  connections:
  Three-Phase V-I Measurementpt_34/LConn1 -- A/RConn1
  Three-Phase V-I Measurementpt_34/RConn1 -- a/RConn1
  Three-Phase V-I Measurementpt_34/LConn2 -- B/RConn1
  Three-Phase V-I Measurementpt_34/LConn3 -- C/RConn1
  Three-Phase V-I Measurementpt_34/RConn3 -- c/RConn1
  Three-Phase V-I Measurementpt_34/RConn2 -- b/RConn1

== system RADTRANS002/M_OUT_Город_3_4 ==
  Iptg_36 : Display
      settings: Format=bank
  PQptg_36 : Scope  NumInputPorts=2
  "Power0 (3ph, Instantaneous)" : powerlib_meascontrol/Measurements/Power (3ph, Instantaneous)
  Pptg_36 : Display
      settings: Format=bank
  Qptg_36 : Display
      settings: Format=bank
  RMS3 : dspstat3/RMS  run=off  directionMode=Each column  dimension=1  InputProcessing=Columns as channels (frame based)  reset_popup=None
  RMS36 : dspstat3/RMS  run=off  directionMode=Each column  dimension=1  InputProcessing=Columns as channels (frame based)  reset_popup=None
  RMS4 : dspstat3/RMS  run=off  directionMode=Each column  dimension=1  InputProcessing=Columns as channels (frame based)  reset_popup=None
  RMSpt_36 : dspstat3/RMS  run=off  directionMode=Each column  dimension=1  InputProcessing=Columns as channels (frame based)  reset_popup=None
  Real-Ima to Complex : RealImagToComplex
  S : Abs
  SSptg_36 : Scope
  Sptg_36 : Display
      settings: Format=bank
  Three-Phase V-I Measurementpt_36 : powerlib/Measurements/Three-Phase V-I Measurement  VoltageMeasurement=phase-to-ground  SetLabelV=off  LabelV=Vabc  Vpu=off  VpuLL=off  CurrentMeasurement=yes  SetLabelI=off  LabelI=Iabc  Ipu=off  Pbase=100e6  Vbase=500e3  OutputType=Complex  PhasorSimulation=off  PSBequivalent=0
  UIptg_36 : Scope  NumInputPorts=2
  Uptg_36 : Display
      settings: Format=bank
  a : PMIOPort  Side=Right
  b : PMIOPort  Port=2  Side=Right
  c : PMIOPort  Port=3  Side=Right
  A : PMIOPort  Port=4  Side=Left
  B : PMIOPort  Port=5  Side=Left
  C : PMIOPort  Port=6  Side=Left
  tag scope: I_ptg_36=global, P_ptg_36=global, Q_ptg_36=global, S_ptg_36=global, U_ptg_36=global
  wires:
  S/1 -> [S_ptg_36]
  Real-Ima to Complex/1 -> S/1
  [S_ptg_36] -> Sptg_36/1
  [S_ptg_36] -> SSptg_36/1
  [P_ptg_36] -> RMSpt_36/1
  RMSpt_36/1 -> Pptg_36/1
  RMS36/1 -> Qptg_36/1
  [U_ptg_36] -> RMS3/1
  RMS3/1 -> Uptg_36/1
  [P_ptg_36] -> Real-Ima to Complex/1
  [Q_ptg_36] -> RMS36/1
  [I_ptg_36] -> RMS4/1
  RMS4/1 -> Iptg_36/1
  [U_ptg_36] -> UIptg_36/1  "U"
  [P_ptg_36] -> PQptg_36/1  "P"
  [I_ptg_36] -> UIptg_36/2  "I"
  Three-Phase V-I Measurementpt_36/1 -> [U_ptg_36]
  [Q_ptg_36] -> Real-Ima to Complex/2
  Three-Phase V-I Measurementpt_36/2 -> [I_ptg_36]
  [U_ptg_36] -> "Power0 (3ph, Instantaneous)"/1
  [I_ptg_36] -> "Power0 (3ph, Instantaneous)"/2
  "Power0 (3ph, Instantaneous)"/2 -> [Q_ptg_36]
  "Power0 (3ph, Instantaneous)"/1 -> [P_ptg_36]
  [Q_ptg_36] -> PQptg_36/2  "Q"
  connections:
  Three-Phase V-I Measurementpt_36/LConn1 -- A/RConn1
  Three-Phase V-I Measurementpt_36/RConn1 -- a/RConn1
  Three-Phase V-I Measurementpt_36/LConn2 -- B/RConn1
  Three-Phase V-I Measurementpt_36/LConn3 -- C/RConn1
  Three-Phase V-I Measurementpt_36/RConn3 -- c/RConn1
  Three-Phase V-I Measurementpt_36/RConn2 -- b/RConn1

== system RADTRANS002/M_OUT_Город_4_1 ==
  Iptg_42 : Display
      settings: Format=bank
  PQptg_42 : Scope  NumInputPorts=2
  "Power0 (3ph, Instantaneous)" : powerlib_meascontrol/Measurements/Power (3ph, Instantaneous)
  Pptg_42 : Display
      settings: Format=bank
  Qptg_42 : Display
      settings: Format=bank
  RMS3 : dspstat3/RMS  run=off  directionMode=Each column  dimension=1  InputProcessing=Columns as channels (frame based)  reset_popup=None
  RMS4 : dspstat3/RMS  run=off  directionMode=Each column  dimension=1  InputProcessing=Columns as channels (frame based)  reset_popup=None
  RMS42 : dspstat3/RMS  run=off  directionMode=Each column  dimension=1  InputProcessing=Columns as channels (frame based)  reset_popup=None
  RMSpt_42 : dspstat3/RMS  run=off  directionMode=Each column  dimension=1  InputProcessing=Columns as channels (frame based)  reset_popup=None
  Real-Ima to Complex : RealImagToComplex
  S : Abs
  SSptg_42 : Scope
  Sptg_42 : Display
      settings: Format=bank
  Three-Phase V-I Measurementpt_42 : powerlib/Measurements/Three-Phase V-I Measurement  VoltageMeasurement=phase-to-ground  SetLabelV=off  LabelV=Vabc  Vpu=off  VpuLL=off  CurrentMeasurement=yes  SetLabelI=off  LabelI=Iabc  Ipu=off  Pbase=100e6  Vbase=500e3  OutputType=Complex  PhasorSimulation=off  PSBequivalent=0
  UIptg_42 : Scope  NumInputPorts=2
  Uptg_42 : Display
      settings: Format=bank
  a : PMIOPort  Side=Right
  b : PMIOPort  Port=2  Side=Right
  c : PMIOPort  Port=3  Side=Right
  A : PMIOPort  Port=4  Side=Left
  B : PMIOPort  Port=5  Side=Left
  C : PMIOPort  Port=6  Side=Left
  tag scope: I_ptg_42=global, P_ptg_42=global, Q_ptg_42=global, S_ptg_42=global, U_ptg_42=global
  wires:
  S/1 -> [S_ptg_42]
  Real-Ima to Complex/1 -> S/1
  [S_ptg_42] -> Sptg_42/1
  [S_ptg_42] -> SSptg_42/1
  [P_ptg_42] -> RMSpt_42/1
  RMSpt_42/1 -> Pptg_42/1
  RMS42/1 -> Qptg_42/1
  [U_ptg_42] -> RMS3/1
  RMS3/1 -> Uptg_42/1
  [P_ptg_42] -> Real-Ima to Complex/1
  [Q_ptg_42] -> RMS42/1
  [I_ptg_42] -> RMS4/1
  RMS4/1 -> Iptg_42/1
  [U_ptg_42] -> UIptg_42/1  "U"
  [P_ptg_42] -> PQptg_42/1  "P"
  [I_ptg_42] -> UIptg_42/2  "I"
  Three-Phase V-I Measurementpt_42/1 -> [U_ptg_42]
  [Q_ptg_42] -> Real-Ima to Complex/2
  Three-Phase V-I Measurementpt_42/2 -> [I_ptg_42]
  [U_ptg_42] -> "Power0 (3ph, Instantaneous)"/1
  [I_ptg_42] -> "Power0 (3ph, Instantaneous)"/2
  "Power0 (3ph, Instantaneous)"/2 -> [Q_ptg_42]
  "Power0 (3ph, Instantaneous)"/1 -> [P_ptg_42]
  [Q_ptg_42] -> PQptg_42/2  "Q"
  connections:
  Three-Phase V-I Measurementpt_42/LConn1 -- A/RConn1
  Three-Phase V-I Measurementpt_42/RConn1 -- a/RConn1
  Three-Phase V-I Measurementpt_42/LConn2 -- B/RConn1
  Three-Phase V-I Measurementpt_42/LConn3 -- C/RConn1
  Three-Phase V-I Measurementpt_42/RConn3 -- c/RConn1
  Three-Phase V-I Measurementpt_42/RConn2 -- b/RConn1

== system RADTRANS002/M_OUT_Город_4_2 ==
  Iptg_44 : Display
      settings: Format=bank
  PQptg_44 : Scope  NumInputPorts=2
  "Power0 (3ph, Instantaneous)" : powerlib_meascontrol/Measurements/Power (3ph, Instantaneous)
  Pptg_44 : Display
      settings: Format=bank
  Qptg_44 : Display
      settings: Format=bank
  RMS3 : dspstat3/RMS  run=off  directionMode=Each column  dimension=1  InputProcessing=Columns as channels (frame based)  reset_popup=None
  RMS4 : dspstat3/RMS  run=off  directionMode=Each column  dimension=1  InputProcessing=Columns as channels (frame based)  reset_popup=None
  RMS44 : dspstat3/RMS  run=off  directionMode=Each column  dimension=1  InputProcessing=Columns as channels (frame based)  reset_popup=None
  RMSpt_44 : dspstat3/RMS  run=off  directionMode=Each column  dimension=1  InputProcessing=Columns as channels (frame based)  reset_popup=None
  Real-Ima to Complex : RealImagToComplex
  S : Abs
  SSptg_44 : Scope
  Sptg_44 : Display
      settings: Format=bank
  Three-Phase V-I Measurementpt_44 : powerlib/Measurements/Three-Phase V-I Measurement  VoltageMeasurement=phase-to-ground  SetLabelV=off  LabelV=Vabc  Vpu=off  VpuLL=off  CurrentMeasurement=yes  SetLabelI=off  LabelI=Iabc  Ipu=off  Pbase=100e6  Vbase=500e3  OutputType=Complex  PhasorSimulation=off  PSBequivalent=0
  UIptg_44 : Scope  NumInputPorts=2
  Uptg_44 : Display
      settings: Format=bank
  a : PMIOPort  Side=Right
  b : PMIOPort  Port=2  Side=Right
  c : PMIOPort  Port=3  Side=Right
  A : PMIOPort  Port=4  Side=Left
  B : PMIOPort  Port=5  Side=Left
  C : PMIOPort  Port=6  Side=Left
  tag scope: I_ptg_44=global, P_ptg_44=global, Q_ptg_44=global, S_ptg_44=global, U_ptg_44=global
  wires:
  S/1 -> [S_ptg_44]
  Real-Ima to Complex/1 -> S/1
  [S_ptg_44] -> Sptg_44/1
  [S_ptg_44] -> SSptg_44/1
  [P_ptg_44] -> RMSpt_44/1
  RMSpt_44/1 -> Pptg_44/1
  RMS44/1 -> Qptg_44/1
  [U_ptg_44] -> RMS3/1
  RMS3/1 -> Uptg_44/1
  [P_ptg_44] -> Real-Ima to Complex/1
  [Q_ptg_44] -> RMS44/1
  [I_ptg_44] -> RMS4/1
  RMS4/1 -> Iptg_44/1
  [U_ptg_44] -> UIptg_44/1  "U"
  [P_ptg_44] -> PQptg_44/1  "P"
  [I_ptg_44] -> UIptg_44/2  "I"
  Three-Phase V-I Measurementpt_44/1 -> [U_ptg_44]
  [Q_ptg_44] -> Real-Ima to Complex/2
  Three-Phase V-I Measurementpt_44/2 -> [I_ptg_44]
  [U_ptg_44] -> "Power0 (3ph, Instantaneous)"/1
  [I_ptg_44] -> "Power0 (3ph, Instantaneous)"/2
  "Power0 (3ph, Instantaneous)"/2 -> [Q_ptg_44]
  "Power0 (3ph, Instantaneous)"/1 -> [P_ptg_44]
  [Q_ptg_44] -> PQptg_44/2  "Q"
  connections:
  Three-Phase V-I Measurementpt_44/LConn1 -- A/RConn1
  Three-Phase V-I Measurementpt_44/RConn1 -- a/RConn1
  Three-Phase V-I Measurementpt_44/LConn2 -- B/RConn1
  Three-Phase V-I Measurementpt_44/LConn3 -- C/RConn1
  Three-Phase V-I Measurementpt_44/RConn3 -- c/RConn1
  Three-Phase V-I Measurementpt_44/RConn2 -- b/RConn1

== system RADTRANS002/M_OUT_Город_4_3 ==
  Iptg_46 : Display
      settings: Format=bank
  PQptg_46 : Scope  NumInputPorts=2
  "Power0 (3ph, Instantaneous)" : powerlib_meascontrol/Measurements/Power (3ph, Instantaneous)
  Pptg_46 : Display
      settings: Format=bank
  Qptg_46 : Display
      settings: Format=bank
  RMS3 : dspstat3/RMS  run=off  directionMode=Each column  dimension=1  InputProcessing=Columns as channels (frame based)  reset_popup=None
  RMS4 : dspstat3/RMS  run=off  directionMode=Each column  dimension=1  InputProcessing=Columns as channels (frame based)  reset_popup=None
  RMS46 : dspstat3/RMS  run=off  directionMode=Each column  dimension=1  InputProcessing=Columns as channels (frame based)  reset_popup=None
  RMSpt_46 : dspstat3/RMS  run=off  directionMode=Each column  dimension=1  InputProcessing=Columns as channels (frame based)  reset_popup=None
  Real-Ima to Complex : RealImagToComplex
  S : Abs
  SSptg_46 : Scope
  Sptg_46 : Display
      settings: Format=bank
  Three-Phase V-I Measurementpt_46 : powerlib/Measurements/Three-Phase V-I Measurement  VoltageMeasurement=phase-to-ground  SetLabelV=off  LabelV=Vabc  Vpu=off  VpuLL=off  CurrentMeasurement=yes  SetLabelI=off  LabelI=Iabc  Ipu=off  Pbase=100e6  Vbase=500e3  OutputType=Complex  PhasorSimulation=off  PSBequivalent=0
  UIptg_46 : Scope  NumInputPorts=2
  Uptg_46 : Display
      settings: Format=bank
  a : PMIOPort  Side=Right
  b : PMIOPort  Port=2  Side=Right
  c : PMIOPort  Port=3  Side=Right
  A : PMIOPort  Port=4  Side=Left
  B : PMIOPort  Port=5  Side=Left
  C : PMIOPort  Port=6  Side=Left
  tag scope: I_ptg_46=global, P_ptg_46=global, Q_ptg_46=global, S_ptg_46=global, U_ptg_46=global
  wires:
  S/1 -> [S_ptg_46]
  Real-Ima to Complex/1 -> S/1
  [S_ptg_46] -> Sptg_46/1
  [S_ptg_46] -> SSptg_46/1
  [P_ptg_46] -> RMSpt_46/1
  RMSpt_46/1 -> Pptg_46/1
  RMS46/1 -> Qptg_46/1
  [U_ptg_46] -> RMS3/1
  RMS3/1 -> Uptg_46/1
  [P_ptg_46] -> Real-Ima to Complex/1
  [Q_ptg_46] -> RMS46/1
  [I_ptg_46] -> RMS4/1
  RMS4/1 -> Iptg_46/1
  [U_ptg_46] -> UIptg_46/1  "U"
  [P_ptg_46] -> PQptg_46/1  "P"
  [I_ptg_46] -> UIptg_46/2  "I"
  Three-Phase V-I Measurementpt_46/1 -> [U_ptg_46]
  [Q_ptg_46] -> Real-Ima to Complex/2
  Three-Phase V-I Measurementpt_46/2 -> [I_ptg_46]
  [U_ptg_46] -> "Power0 (3ph, Instantaneous)"/1
  [I_ptg_46] -> "Power0 (3ph, Instantaneous)"/2
  "Power0 (3ph, Instantaneous)"/2 -> [Q_ptg_46]
  "Power0 (3ph, Instantaneous)"/1 -> [P_ptg_46]
  [Q_ptg_46] -> PQptg_46/2  "Q"
  connections:
  Three-Phase V-I Measurementpt_46/LConn1 -- A/RConn1
  Three-Phase V-I Measurementpt_46/RConn1 -- a/RConn1
  Three-Phase V-I Measurementpt_46/LConn2 -- B/RConn1
  Three-Phase V-I Measurementpt_46/LConn3 -- C/RConn1
  Three-Phase V-I Measurementpt_46/RConn3 -- c/RConn1
  Three-Phase V-I Measurementpt_46/RConn2 -- b/RConn1
